simulink model "Base_Map_cs"  (R2019a)
settings: Solver=FixedStepDiscrete  StartTime=0.0  StopTime=15  FixedStep=1/300  RelTol=1e-3
PreLoadFcn:
  | mbxruntime.callbacks.PreLoadFcn(bdroot);
  | check_NUTS_defined
  | model_closed = 0;
  | assignin('base',['model_closed_' bdroot],false);
PostLoadFcn:
  | mbxruntime.callbacks.PostLoadFcn(bdroot);
InitFcn:
  | mbxruntime.callbacks.InitFcn(bdroot);
StartFcn:
  | mbxruntime.callbacks.StartFcn(bdroot);
StopFcn:
  | mbxruntime.callbacks.StopFcn(bdroot);;
  | 
model workspace: external: MAT-File .\Base_Map_S_cs_hws.mat (data not in the file)
undefined symbols (not defined in the file or in its folder): AngularVelocity, Clock_, Data, Data_SL_Info, DiscIntNeverNeededParam, Encoding, Encoding_SL_Info, Header, Height, InitImageOutputDir, LinearAcceleration, mbxruntime, Orientation, Pose, Poses, Poses_SL_Info, Position, Step, tabledata, Twist, Width
libraries: PBCSimulinkLibrary x53, robotlib x26, simulink_extras x19, PreScanSimulinkLibrary x6, dspindex x4, robotcorelib x2, sharedtransform x2, visionconversions x1, visionsinks x1
(part 4 of 8)

== system Base_Map_cs/TrafficLightRoadSideNL_5_Casing.LightOrange_Control ==
  TrafficLightRoadSideNL_5_Casing.LightOrange_Control : Inport  Tag=inport/plugin/sfun_PBCLight  OutDataTypeStr=Bus: PRESCAN_PBCLIGHT_DATA  PortDimensions=1  SampleTime=0.05  BusOutputAsStruct=on
  Actuator : S-Function  LoadFcn=addpath 'C:/Program Files/Simcenter Prescan/Prescan_2019.1/Plugins/PBCameraPlugin/matlab';addpath 'C:/Program Files/Simcenter Prescan/Prescan_2019.1/Plugins/PBCameraPlugin/bin';load('PreScanPBCLightData.mat');  FunctionName=sfun_PBCLight  Parameters=lightID, timestepMask  SFunctionDeploymentMode=off  EnableBusSupport=off  mask(Physics Based Camera plugin block){lightID=13, timestepMask=0.05}
      mask prompts: lightID "Light ID:"; timestepMask "MATLAB timestep:"
      mask help: Light Control I/O
      mask Help: eval('openHelp(6500)')
      mask Display: image(imread('ico_PBCControl.png'))
  wires:
  TrafficLightRoadSideNL_5_Casing.LightOrange_Control/1 -> Actuator/1

== system Base_Map_cs/TrafficLightRoadSideNL_5_Casing.LightRed_Control ==
  TrafficLightRoadSideNL_5_Casing.LightRed_Control : Inport  Tag=inport/plugin/sfun_PBCLight  OutDataTypeStr=Bus: PRESCAN_PBCLIGHT_DATA  PortDimensions=1  SampleTime=0.05  BusOutputAsStruct=on
  Actuator : S-Function  LoadFcn=addpath 'C:/Program Files/Simcenter Prescan/Prescan_2019.1/Plugins/PBCameraPlugin/matlab';addpath 'C:/Program Files/Simcenter Prescan/Prescan_2019.1/Plugins/PBCameraPlugin/bin';load('PreScanPBCLightData.mat');  FunctionName=sfun_PBCLight  Parameters=lightID, timestepMask  SFunctionDeploymentMode=off  EnableBusSupport=off  mask(Physics Based Camera plugin block){lightID=12, timestepMask=0.05}
      mask prompts: lightID "Light ID:"; timestepMask "MATLAB timestep:"
      mask help: Light Control I/O
      mask Help: eval('openHelp(6500)')
      mask Display: image(imread('ico_PBCControl.png'))
  wires:
  TrafficLightRoadSideNL_5_Casing.LightRed_Control/1 -> Actuator/1

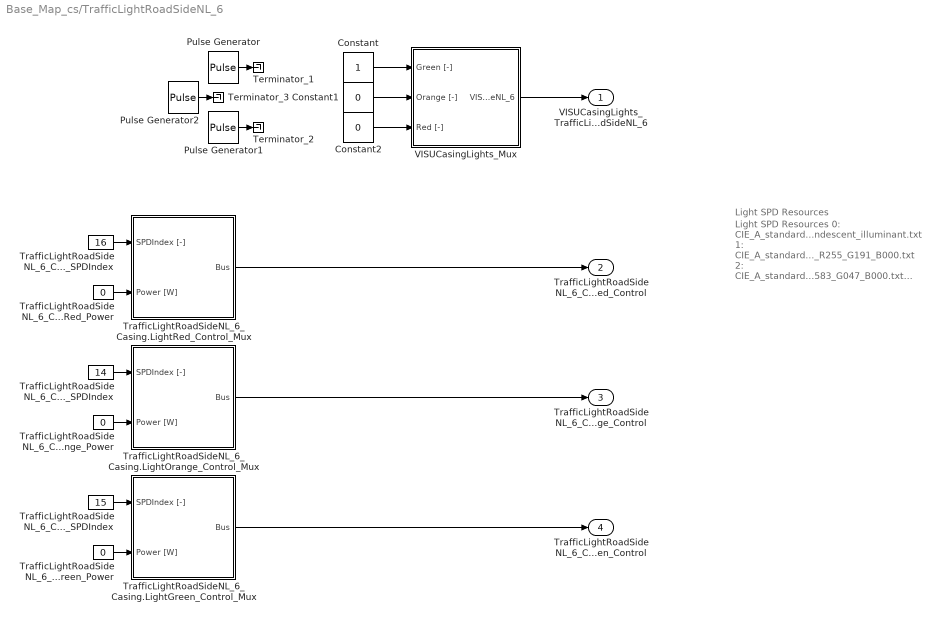
== system Base_Map_cs/TrafficLightRoadSideNL_6 ==
  note: Light SPD Resources
      |
      |  0: CIE_A_standard_incandescent_illuminant.txt
      |  1: CIE_A_standard_incandescent_illuminant.txt_x_R255_G191_B000.txt
      |  2: CIE_A_standard_incandescent_illuminant.txt_x_R583_G047_B000.txt
      |  3: CIE_F12_standard_fluorescent_illuminant.txt
      |  4: Illuminant_D65.txt
      |  5: Light_SPD_H1_12_8V_Filament.txt
      |  6: Light_SPD_H1_13_2V_Filament.txt
      |  7: Light_SPD_H11_12V_Filament.txt
      |  8: Light_SPD_H7_12_8V_Filament.txt
      |  9: Light_SPD_H7_13_2V_Filament.txt
      | 10: Light_SPD_H8_13_2V_Filament.txt
      | 11: Light_SPD_Halogen.txt
      | 12: Light_SPD_High_Power_LED.txt
      | 13: Light_SPD_HPS_High_Pressure_Sodium.txt
      | 14: Light_SPD_incandescent_traffic_signal_amber.txt
      | 15: Light_SPD_incandescent_traffic_signal_green.txt
      | 16: Light_SPD_incandescent_traffic_signal_red.txt
      | 17: Light_SPD_LED_D1S_HID.txt
      | 18: Light_SPD_LED_traffic_signal_amber.txt
      | 19: Light_SPD_LED_traffic_signal_green.txt
      | 20: Light_SPD_LED_traffic_signal_red.txt
      | 21: Light_SPD_LPS_Low_Pressure_Sodium.txt
      | 22: Light_SPD_Mercury.txt
      | 23: Light_SPD_Reddish_Neon_Sign.txt
      | 24: Noma_Twister_Blue_13W_120V.txt
      | 25: Philips_Blue_Golite_P1_Apollo_1750Lux.txt
      | 26: SPD_flat_1.0.txt
  note: Light SPD Resources
  Constant : Constant
  Constant1 : Constant  Value=0
  Constant2 : Constant  Value=0
  Pulse Generator : DiscretePulseGenerator  PulseType=Time based  Period=10  PulseWidth=40
  Pulse Generator1 : DiscretePulseGenerator  PulseType=Time based  Period=10  PulseWidth=40  PhaseDelay=6
  Pulse Generator2 : DiscretePulseGenerator  PulseType=Time based  Period=10  PulseWidth=20  PhaseDelay=4
  Terminator_1 : Terminator
  Terminator_2 : Terminator
  Terminator_3 : Terminator
  TrafficLightRoadSideNL_6_Casing.LightGreen_Control_Mux : Subsystem  Tag=mux/plugin/LightSignals
  TrafficLightRoadSideNL_6_Casing.LightGreen_Power : Constant  Tag=TrafficLightRoadSideNL_6_Casing.LightGreen_Power  Value=0
  TrafficLightRoadSideNL_6_Casing.LightGreen_SPDIndex : Constant  Tag=TrafficLightRoadSideNL_6_Casing.LightGreen_SPDIndex  Value=15
  TrafficLightRoadSideNL_6_Casing.LightOrange_Control_Mux : Subsystem  Tag=mux/plugin/LightSignals
  TrafficLightRoadSideNL_6_Casing.LightOrange_Power : Constant  Tag=TrafficLightRoadSideNL_6_Casing.LightOrange_Power  Value=0
  TrafficLightRoadSideNL_6_Casing.LightOrange_SPDIndex : Constant  Tag=TrafficLightRoadSideNL_6_Casing.LightOrange_SPDIndex  Value=14
  TrafficLightRoadSideNL_6_Casing.LightRed_Control_Mux : Subsystem  Tag=mux/plugin/LightSignals
  TrafficLightRoadSideNL_6_Casing.LightRed_Power : Constant  Tag=TrafficLightRoadSideNL_6_Casing.LightRed_Power  Value=0
  TrafficLightRoadSideNL_6_Casing.LightRed_SPDIndex : Constant  Tag=TrafficLightRoadSideNL_6_Casing.LightRed_SPDIndex  Value=16
  VISUCasingLights_Mux : Subsystem  Tag=mux/VisuCasingLights  mask(PreScan User Interface: VisuTrafficLight){}
      mask help:
      | The VisuTrafficLight block provides a way to animate traffic lights: switch on and off individual lights.
      |
      | For more information, please click Help.
      mask Help: eval('openHelp(731)')
  VISUCasingLights_TrafficLightRoadSideNL_6 : Outport  Tag=outport/VisuCasingLights  SampleTime=1/300
  TrafficLightRoadSideNL_6_Casing.LightRed_Control : Outport  Tag=outport/plugin/sfun_PBCLight  Port=2  OutDataTypeStr=Bus: PRESCAN_PBCLIGHT_DATA  PortDimensions=1  SampleTime=0.05
  TrafficLightRoadSideNL_6_Casing.LightOrange_Control : Outport  Tag=outport/plugin/sfun_PBCLight  Port=3  OutDataTypeStr=Bus: PRESCAN_PBCLIGHT_DATA  PortDimensions=1  SampleTime=0.05
  TrafficLightRoadSideNL_6_Casing.LightGreen_Control : Outport  Tag=outport/plugin/sfun_PBCLight  Port=4  OutDataTypeStr=Bus: PRESCAN_PBCLIGHT_DATA  PortDimensions=1  SampleTime=0.05
  wires:
  Constant/1 -> VISUCasingLights_Mux/1(Green [-])
  Constant1/1 -> VISUCasingLights_Mux/2(Orange [-])
  Constant2/1 -> VISUCasingLights_Mux/3(Red [-])
  VISUCasingLights_Mux/1(VISUCasingLights_TrafficLightRoadSideNL_6) -> VISUCasingLights_TrafficLightRoadSideNL_6/1
  TrafficLightRoadSideNL_6_Casing.LightRed_Control_Mux/1(Bus) -> TrafficLightRoadSideNL_6_Casing.LightRed_Control/1
  TrafficLightRoadSideNL_6_Casing.LightRed_SPDIndex/1 -> TrafficLightRoadSideNL_6_Casing.LightRed_Control_Mux/1(SPDIndex [-])
  TrafficLightRoadSideNL_6_Casing.LightRed_Power/1 -> TrafficLightRoadSideNL_6_Casing.LightRed_Control_Mux/2(Power [W])
  TrafficLightRoadSideNL_6_Casing.LightOrange_Control_Mux/1(Bus) -> TrafficLightRoadSideNL_6_Casing.LightOrange_Control/1
  TrafficLightRoadSideNL_6_Casing.LightOrange_SPDIndex/1 -> TrafficLightRoadSideNL_6_Casing.LightOrange_Control_Mux/1(SPDIndex [-])
  TrafficLightRoadSideNL_6_Casing.LightOrange_Power/1 -> TrafficLightRoadSideNL_6_Casing.LightOrange_Control_Mux/2(Power [W])
  TrafficLightRoadSideNL_6_Casing.LightGreen_Control_Mux/1(Bus) -> TrafficLightRoadSideNL_6_Casing.LightGreen_Control/1
  TrafficLightRoadSideNL_6_Casing.LightGreen_SPDIndex/1 -> TrafficLightRoadSideNL_6_Casing.LightGreen_Control_Mux/1(SPDIndex [-])
  TrafficLightRoadSideNL_6_Casing.LightGreen_Power/1 -> TrafficLightRoadSideNL_6_Casing.LightGreen_Control_Mux/2(Power [W])
  Pulse Generator/1 -> Terminator_1/1
  Pulse Generator1/1 -> Terminator_2/1
  Pulse Generator2/1 -> Terminator_3/1

== system Base_Map_cs/TrafficLightRoadSideNL_6_Casing.LightGreen_Control ==
  TrafficLightRoadSideNL_6_Casing.LightGreen_Control : Inport  Tag=inport/plugin/sfun_PBCLight  OutDataTypeStr=Bus: PRESCAN_PBCLIGHT_DATA  PortDimensions=1  SampleTime=0.05  BusOutputAsStruct=on
  Actuator : S-Function  LoadFcn=addpath 'C:/Program Files/Simcenter Prescan/Prescan_2019.1/Plugins/PBCameraPlugin/matlab';addpath 'C:/Program Files/Simcenter Prescan/Prescan_2019.1/Plugins/PBCameraPlugin/bin';load('PreScanPBCLightData.mat');  FunctionName=sfun_PBCLight  Parameters=lightID, timestepMask  SFunctionDeploymentMode=off  EnableBusSupport=off  mask(Physics Based Camera plugin block){lightID=23, timestepMask=0.05}
      mask prompts: lightID "Light ID:"; timestepMask "MATLAB timestep:"
      mask help: Light Control I/O
      mask Help: eval('openHelp(6500)')
      mask Display: image(imread('ico_PBCControl.png'))
  wires:
  TrafficLightRoadSideNL_6_Casing.LightGreen_Control/1 -> Actuator/1

== system Base_Map_cs/TrafficLightRoadSideNL_6_Casing.LightOrange_Control ==
  TrafficLightRoadSideNL_6_Casing.LightOrange_Control : Inport  Tag=inport/plugin/sfun_PBCLight  OutDataTypeStr=Bus: PRESCAN_PBCLIGHT_DATA  PortDimensions=1  SampleTime=0.05  BusOutputAsStruct=on
  Actuator : S-Function  LoadFcn=addpath 'C:/Program Files/Simcenter Prescan/Prescan_2019.1/Plugins/PBCameraPlugin/matlab';addpath 'C:/Program Files/Simcenter Prescan/Prescan_2019.1/Plugins/PBCameraPlugin/bin';load('PreScanPBCLightData.mat');  FunctionName=sfun_PBCLight  Parameters=lightID, timestepMask  SFunctionDeploymentMode=off  EnableBusSupport=off  mask(Physics Based Camera plugin block){lightID=22, timestepMask=0.05}
      mask prompts: lightID "Light ID:"; timestepMask "MATLAB timestep:"
      mask help: Light Control I/O
      mask Help: eval('openHelp(6500)')
      mask Display: image(imread('ico_PBCControl.png'))
  wires:
  TrafficLightRoadSideNL_6_Casing.LightOrange_Control/1 -> Actuator/1

== system Base_Map_cs/TrafficLightRoadSideNL_6_Casing.LightRed_Control ==
  TrafficLightRoadSideNL_6_Casing.LightRed_Control : Inport  Tag=inport/plugin/sfun_PBCLight  OutDataTypeStr=Bus: PRESCAN_PBCLIGHT_DATA  PortDimensions=1  SampleTime=0.05  BusOutputAsStruct=on
  Actuator : S-Function  LoadFcn=addpath 'C:/Program Files/Simcenter Prescan/Prescan_2019.1/Plugins/PBCameraPlugin/matlab';addpath 'C:/Program Files/Simcenter Prescan/Prescan_2019.1/Plugins/PBCameraPlugin/bin';load('PreScanPBCLightData.mat');  FunctionName=sfun_PBCLight  Parameters=lightID, timestepMask  SFunctionDeploymentMode=off  EnableBusSupport=off  mask(Physics Based Camera plugin block){lightID=21, timestepMask=0.05}
      mask prompts: lightID "Light ID:"; timestepMask "MATLAB timestep:"
      mask help: Light Control I/O
      mask Help: eval('openHelp(6500)')
      mask Display: image(imread('ico_PBCControl.png'))
  wires:
  TrafficLightRoadSideNL_6_Casing.LightRed_Control/1 -> Actuator/1

== system Base_Map_cs/TrafficLightRoadSideNL_7 ==
  note: Light SPD Resources
      |
      |  0: CIE_A_standard_incandescent_illuminant.txt
      |  1: CIE_A_standard_incandescent_illuminant.txt_x_R255_G191_B000.txt
      |  2: CIE_A_standard_incandescent_illuminant.txt_x_R583_G047_B000.txt
      |  3: CIE_F12_standard_fluorescent_illuminant.txt
      |  4: Illuminant_D65.txt
      |  5: Light_SPD_H1_12_8V_Filament.txt
      |  6: Light_SPD_H1_13_2V_Filament.txt
      |  7: Light_SPD_H11_12V_Filament.txt
      |  8: Light_SPD_H7_12_8V_Filament.txt
      |  9: Light_SPD_H7_13_2V_Filament.txt
      | 10: Light_SPD_H8_13_2V_Filament.txt
      | 11: Light_SPD_Halogen.txt
      | 12: Light_SPD_High_Power_LED.txt
      | 13: Light_SPD_HPS_High_Pressure_Sodium.txt
      | 14: Light_SPD_incandescent_traffic_signal_amber.txt
      | 15: Light_SPD_incandescent_traffic_signal_green.txt
      | 16: Light_SPD_incandescent_traffic_signal_red.txt
      | 17: Light_SPD_LED_D1S_HID.txt
      | 18: Light_SPD_LED_traffic_signal_amber.txt
      | 19: Light_SPD_LED_traffic_signal_green.txt
      | 20: Light_SPD_LED_traffic_signal_red.txt
      | 21: Light_SPD_LPS_Low_Pressure_Sodium.txt
      | 22: Light_SPD_Mercury.txt
      | 23: Light_SPD_Reddish_Neon_Sign.txt
      | 24: Noma_Twister_Blue_13W_120V.txt
      | 25: Philips_Blue_Golite_P1_Apollo_1750Lux.txt
      | 26: SPD_flat_1.0.txt
  note: Light SPD Resources
  Ground_1 : Ground
  Ground_2 : Ground
  Ground_3 : Ground
  TrafficLightRoadSideNL_7_Casing.LightGreen_Control_Mux : Subsystem  Tag=mux/plugin/LightSignals
  TrafficLightRoadSideNL_7_Casing.LightGreen_Power : Constant  Tag=TrafficLightRoadSideNL_7_Casing.LightGreen_Power  Value=0
  TrafficLightRoadSideNL_7_Casing.LightGreen_SPDIndex : Constant  Tag=TrafficLightRoadSideNL_7_Casing.LightGreen_SPDIndex  Value=15
  TrafficLightRoadSideNL_7_Casing.LightOrange_Control_Mux : Subsystem  Tag=mux/plugin/LightSignals
  TrafficLightRoadSideNL_7_Casing.LightOrange_Power : Constant  Tag=TrafficLightRoadSideNL_7_Casing.LightOrange_Power  Value=0
  TrafficLightRoadSideNL_7_Casing.LightOrange_SPDIndex : Constant  Tag=TrafficLightRoadSideNL_7_Casing.LightOrange_SPDIndex  Value=14
  TrafficLightRoadSideNL_7_Casing.LightRed_Control_Mux : Subsystem  Tag=mux/plugin/LightSignals
  TrafficLightRoadSideNL_7_Casing.LightRed_Power : Constant  Tag=TrafficLightRoadSideNL_7_Casing.LightRed_Power  Value=0
  TrafficLightRoadSideNL_7_Casing.LightRed_SPDIndex : Constant  Tag=TrafficLightRoadSideNL_7_Casing.LightRed_SPDIndex  Value=16
  VISUCasingLights_Mux : Subsystem  Tag=mux/VisuCasingLights  mask(PreScan User Interface: VisuTrafficLight){}
      mask help:
      | The VisuTrafficLight block provides a way to animate traffic lights: switch on and off individual lights.
      |
      | For more information, please click Help.
      mask Help: eval('openHelp(731)')
  VISUCasingLights_TrafficLightRoadSideNL_7 : Outport  Tag=outport/VisuCasingLights  SampleTime=1/300
  TrafficLightRoadSideNL_7_Casing.LightRed_Control : Outport  Tag=outport/plugin/sfun_PBCLight  Port=2  OutDataTypeStr=Bus: PRESCAN_PBCLIGHT_DATA  PortDimensions=1  SampleTime=0.05
  TrafficLightRoadSideNL_7_Casing.LightOrange_Control : Outport  Tag=outport/plugin/sfun_PBCLight  Port=3  OutDataTypeStr=Bus: PRESCAN_PBCLIGHT_DATA  PortDimensions=1  SampleTime=0.05
  TrafficLightRoadSideNL_7_Casing.LightGreen_Control : Outport  Tag=outport/plugin/sfun_PBCLight  Port=4  OutDataTypeStr=Bus: PRESCAN_PBCLIGHT_DATA  PortDimensions=1  SampleTime=0.05
  wires:
  VISUCasingLights_Mux/1(VISUCasingLights_TrafficLightRoadSideNL_7) -> VISUCasingLights_TrafficLightRoadSideNL_7/1
  TrafficLightRoadSideNL_7_Casing.LightRed_Control_Mux/1(Bus) -> TrafficLightRoadSideNL_7_Casing.LightRed_Control/1
  TrafficLightRoadSideNL_7_Casing.LightRed_SPDIndex/1 -> TrafficLightRoadSideNL_7_Casing.LightRed_Control_Mux/1(SPDIndex [-])
  TrafficLightRoadSideNL_7_Casing.LightRed_Power/1 -> TrafficLightRoadSideNL_7_Casing.LightRed_Control_Mux/2(Power [W])
  TrafficLightRoadSideNL_7_Casing.LightOrange_Control_Mux/1(Bus) -> TrafficLightRoadSideNL_7_Casing.LightOrange_Control/1
  TrafficLightRoadSideNL_7_Casing.LightOrange_SPDIndex/1 -> TrafficLightRoadSideNL_7_Casing.LightOrange_Control_Mux/1(SPDIndex [-])
  TrafficLightRoadSideNL_7_Casing.LightOrange_Power/1 -> TrafficLightRoadSideNL_7_Casing.LightOrange_Control_Mux/2(Power [W])
  TrafficLightRoadSideNL_7_Casing.LightGreen_Control_Mux/1(Bus) -> TrafficLightRoadSideNL_7_Casing.LightGreen_Control/1
  TrafficLightRoadSideNL_7_Casing.LightGreen_SPDIndex/1 -> TrafficLightRoadSideNL_7_Casing.LightGreen_Control_Mux/1(SPDIndex [-])
  TrafficLightRoadSideNL_7_Casing.LightGreen_Power/1 -> TrafficLightRoadSideNL_7_Casing.LightGreen_Control_Mux/2(Power [W])
  Ground_1/1 -> VISUCasingLights_Mux/1(Green [-])
  Ground_2/1 -> VISUCasingLights_Mux/2(Orange [-])
  Ground_3/1 -> VISUCasingLights_Mux/3(Red [-])

== system Base_Map_cs/TrafficLightRoadSideNL_7_Casing.LightGreen_Control ==
  TrafficLightRoadSideNL_7_Casing.LightGreen_Control : Inport  Tag=inport/plugin/sfun_PBCLight  OutDataTypeStr=Bus: PRESCAN_PBCLIGHT_DATA  PortDimensions=1  SampleTime=0.05  BusOutputAsStruct=on
  Actuator : S-Function  LoadFcn=addpath 'C:/Program Files/Simcenter Prescan/Prescan_2019.1/Plugins/PBCameraPlugin/matlab';addpath 'C:/Program Files/Simcenter Prescan/Prescan_2019.1/Plugins/PBCameraPlugin/bin';load('PreScanPBCLightData.mat');  FunctionName=sfun_PBCLight  Parameters=lightID, timestepMask  SFunctionDeploymentMode=off  EnableBusSupport=off  mask(Physics Based Camera plugin block){lightID=17, timestepMask=0.05}
      mask prompts: lightID "Light ID:"; timestepMask "MATLAB timestep:"
      mask help: Light Control I/O
      mask Help: eval('openHelp(6500)')
      mask Display: image(imread('ico_PBCControl.png'))
  wires:
  TrafficLightRoadSideNL_7_Casing.LightGreen_Control/1 -> Actuator/1

== system Base_Map_cs/TrafficLightRoadSideNL_7_Casing.LightOrange_Control ==
  TrafficLightRoadSideNL_7_Casing.LightOrange_Control : Inport  Tag=inport/plugin/sfun_PBCLight  OutDataTypeStr=Bus: PRESCAN_PBCLIGHT_DATA  PortDimensions=1  SampleTime=0.05  BusOutputAsStruct=on
  Actuator : S-Function  LoadFcn=addpath 'C:/Program Files/Simcenter Prescan/Prescan_2019.1/Plugins/PBCameraPlugin/matlab';addpath 'C:/Program Files/Simcenter Prescan/Prescan_2019.1/Plugins/PBCameraPlugin/bin';load('PreScanPBCLightData.mat');  FunctionName=sfun_PBCLight  Parameters=lightID, timestepMask  SFunctionDeploymentMode=off  EnableBusSupport=off  mask(Physics Based Camera plugin block){lightID=16, timestepMask=0.05}
      mask prompts: lightID "Light ID:"; timestepMask "MATLAB timestep:"
      mask help: Light Control I/O
      mask Help: eval('openHelp(6500)')
      mask Display: image(imread('ico_PBCControl.png'))
  wires:
  TrafficLightRoadSideNL_7_Casing.LightOrange_Control/1 -> Actuator/1

== system Base_Map_cs/TrafficLightRoadSideNL_7_Casing.LightRed_Control ==
  TrafficLightRoadSideNL_7_Casing.LightRed_Control : Inport  Tag=inport/plugin/sfun_PBCLight  OutDataTypeStr=Bus: PRESCAN_PBCLIGHT_DATA  PortDimensions=1  SampleTime=0.05  BusOutputAsStruct=on
  Actuator : S-Function  LoadFcn=addpath 'C:/Program Files/Simcenter Prescan/Prescan_2019.1/Plugins/PBCameraPlugin/matlab';addpath 'C:/Program Files/Simcenter Prescan/Prescan_2019.1/Plugins/PBCameraPlugin/bin';load('PreScanPBCLightData.mat');  FunctionName=sfun_PBCLight  Parameters=lightID, timestepMask  SFunctionDeploymentMode=off  EnableBusSupport=off  mask(Physics Based Camera plugin block){lightID=15, timestepMask=0.05}
      mask prompts: lightID "Light ID:"; timestepMask "MATLAB timestep:"
      mask help: Light Control I/O
      mask Help: eval('openHelp(6500)')
      mask Display: image(imread('ico_PBCControl.png'))
  wires:
  TrafficLightRoadSideNL_7_Casing.LightRed_Control/1 -> Actuator/1

== system Base_Map_cs/TrafficLightRoadSideNL_8 ==
  note: Light SPD Resources
      |
      |  0: CIE_A_standard_incandescent_illuminant.txt
      |  1: CIE_A_standard_incandescent_illuminant.txt_x_R255_G191_B000.txt
      |  2: CIE_A_standard_incandescent_illuminant.txt_x_R583_G047_B000.txt
      |  3: CIE_F12_standard_fluorescent_illuminant.txt
      |  4: Illuminant_D65.txt
      |  5: Light_SPD_H1_12_8V_Filament.txt
      |  6: Light_SPD_H1_13_2V_Filament.txt
      |  7: Light_SPD_H11_12V_Filament.txt
      |  8: Light_SPD_H7_12_8V_Filament.txt
      |  9: Light_SPD_H7_13_2V_Filament.txt
      | 10: Light_SPD_H8_13_2V_Filament.txt
      | 11: Light_SPD_Halogen.txt
      | 12: Light_SPD_High_Power_LED.txt
      | 13: Light_SPD_HPS_High_Pressure_Sodium.txt
      | 14: Light_SPD_incandescent_traffic_signal_amber.txt
      | 15: Light_SPD_incandescent_traffic_signal_green.txt
      | 16: Light_SPD_incandescent_traffic_signal_red.txt
      | 17: Light_SPD_LED_D1S_HID.txt
      | 18: Light_SPD_LED_traffic_signal_amber.txt
      | 19: Light_SPD_LED_traffic_signal_green.txt
      | 20: Light_SPD_LED_traffic_signal_red.txt
      | 21: Light_SPD_LPS_Low_Pressure_Sodium.txt
      | 22: Light_SPD_Mercury.txt
      | 23: Light_SPD_Reddish_Neon_Sign.txt
      | 24: Noma_Twister_Blue_13W_120V.txt
      | 25: Philips_Blue_Golite_P1_Apollo_1750Lux.txt
      | 26: SPD_flat_1.0.txt
  note: Light SPD Resources
  Ground_1 : Ground
  Ground_2 : Ground
  Ground_3 : Ground
  TrafficLightRoadSideNL_8_Casing.LightGreen_Control_Mux : Subsystem  Tag=mux/plugin/LightSignals
  TrafficLightRoadSideNL_8_Casing.LightGreen_Power : Constant  Tag=TrafficLightRoadSideNL_8_Casing.LightGreen_Power  Value=0
  TrafficLightRoadSideNL_8_Casing.LightGreen_SPDIndex : Constant  Tag=TrafficLightRoadSideNL_8_Casing.LightGreen_SPDIndex  Value=15
  TrafficLightRoadSideNL_8_Casing.LightOrange_Control_Mux : Subsystem  Tag=mux/plugin/LightSignals
  TrafficLightRoadSideNL_8_Casing.LightOrange_Power : Constant  Tag=TrafficLightRoadSideNL_8_Casing.LightOrange_Power  Value=0
  TrafficLightRoadSideNL_8_Casing.LightOrange_SPDIndex : Constant  Tag=TrafficLightRoadSideNL_8_Casing.LightOrange_SPDIndex  Value=14
  TrafficLightRoadSideNL_8_Casing.LightRed_Control_Mux : Subsystem  Tag=mux/plugin/LightSignals
  TrafficLightRoadSideNL_8_Casing.LightRed_Power : Constant  Tag=TrafficLightRoadSideNL_8_Casing.LightRed_Power  Value=0
  TrafficLightRoadSideNL_8_Casing.LightRed_SPDIndex : Constant  Tag=TrafficLightRoadSideNL_8_Casing.LightRed_SPDIndex  Value=16
  VISUCasingLights_Mux : Subsystem  Tag=mux/VisuCasingLights  mask(PreScan User Interface: VisuTrafficLight){}
      mask help:
      | The VisuTrafficLight block provides a way to animate traffic lights: switch on and off individual lights.
      |
      | For more information, please click Help.
      mask Help: eval('openHelp(731)')
  VISUCasingLights_TrafficLightRoadSideNL_8 : Outport  Tag=outport/VisuCasingLights  SampleTime=1/300
  TrafficLightRoadSideNL_8_Casing.LightRed_Control : Outport  Tag=outport/plugin/sfun_PBCLight  Port=2  OutDataTypeStr=Bus: PRESCAN_PBCLIGHT_DATA  PortDimensions=1  SampleTime=0.05
  TrafficLightRoadSideNL_8_Casing.LightOrange_Control : Outport  Tag=outport/plugin/sfun_PBCLight  Port=3  OutDataTypeStr=Bus: PRESCAN_PBCLIGHT_DATA  PortDimensions=1  SampleTime=0.05
  TrafficLightRoadSideNL_8_Casing.LightGreen_Control : Outport  Tag=outport/plugin/sfun_PBCLight  Port=4  OutDataTypeStr=Bus: PRESCAN_PBCLIGHT_DATA  PortDimensions=1  SampleTime=0.05
  wires:
  VISUCasingLights_Mux/1(VISUCasingLights_TrafficLightRoadSideNL_8) -> VISUCasingLights_TrafficLightRoadSideNL_8/1
  TrafficLightRoadSideNL_8_Casing.LightRed_Control_Mux/1(Bus) -> TrafficLightRoadSideNL_8_Casing.LightRed_Control/1
  TrafficLightRoadSideNL_8_Casing.LightRed_SPDIndex/1 -> TrafficLightRoadSideNL_8_Casing.LightRed_Control_Mux/1(SPDIndex [-])
  TrafficLightRoadSideNL_8_Casing.LightRed_Power/1 -> TrafficLightRoadSideNL_8_Casing.LightRed_Control_Mux/2(Power [W])
  TrafficLightRoadSideNL_8_Casing.LightOrange_Control_Mux/1(Bus) -> TrafficLightRoadSideNL_8_Casing.LightOrange_Control/1
  TrafficLightRoadSideNL_8_Casing.LightOrange_SPDIndex/1 -> TrafficLightRoadSideNL_8_Casing.LightOrange_Control_Mux/1(SPDIndex [-])
  TrafficLightRoadSideNL_8_Casing.LightOrange_Power/1 -> TrafficLightRoadSideNL_8_Casing.LightOrange_Control_Mux/2(Power [W])
  TrafficLightRoadSideNL_8_Casing.LightGreen_Control_Mux/1(Bus) -> TrafficLightRoadSideNL_8_Casing.LightGreen_Control/1
  TrafficLightRoadSideNL_8_Casing.LightGreen_SPDIndex/1 -> TrafficLightRoadSideNL_8_Casing.LightGreen_Control_Mux/1(SPDIndex [-])
  TrafficLightRoadSideNL_8_Casing.LightGreen_Power/1 -> TrafficLightRoadSideNL_8_Casing.LightGreen_Control_Mux/2(Power [W])
  Ground_1/1 -> VISUCasingLights_Mux/1(Green [-])
  Ground_2/1 -> VISUCasingLights_Mux/2(Orange [-])
  Ground_3/1 -> VISUCasingLights_Mux/3(Red [-])

== system Base_Map_cs/TrafficLightRoadSideNL_8_Casing.LightGreen_Control ==
  TrafficLightRoadSideNL_8_Casing.LightGreen_Control : Inport  Tag=inport/plugin/sfun_PBCLight  OutDataTypeStr=Bus: PRESCAN_PBCLIGHT_DATA  PortDimensions=1  SampleTime=0.05  BusOutputAsStruct=on
  Actuator : S-Function  LoadFcn=addpath 'C:/Program Files/Simcenter Prescan/Prescan_2019.1/Plugins/PBCameraPlugin/matlab';addpath 'C:/Program Files/Simcenter Prescan/Prescan_2019.1/Plugins/PBCameraPlugin/bin';load('PreScanPBCLightData.mat');  FunctionName=sfun_PBCLight  Parameters=lightID, timestepMask  SFunctionDeploymentMode=off  EnableBusSupport=off  mask(Physics Based Camera plugin block){lightID=20, timestepMask=0.05}
      mask prompts: lightID "Light ID:"; timestepMask "MATLAB timestep:"
      mask help: Light Control I/O
      mask Help: eval('openHelp(6500)')
      mask Display: image(imread('ico_PBCControl.png'))
  wires:
  TrafficLightRoadSideNL_8_Casing.LightGreen_Control/1 -> Actuator/1

== system Base_Map_cs/TrafficLightRoadSideNL_8_Casing.LightOrange_Control ==
  TrafficLightRoadSideNL_8_Casing.LightOrange_Control : Inport  Tag=inport/plugin/sfun_PBCLight  OutDataTypeStr=Bus: PRESCAN_PBCLIGHT_DATA  PortDimensions=1  SampleTime=0.05  BusOutputAsStruct=on
  Actuator : S-Function  LoadFcn=addpath 'C:/Program Files/Simcenter Prescan/Prescan_2019.1/Plugins/PBCameraPlugin/matlab';addpath 'C:/Program Files/Simcenter Prescan/Prescan_2019.1/Plugins/PBCameraPlugin/bin';load('PreScanPBCLightData.mat');  FunctionName=sfun_PBCLight  Parameters=lightID, timestepMask  SFunctionDeploymentMode=off  EnableBusSupport=off  mask(Physics Based Camera plugin block){lightID=19, timestepMask=0.05}
      mask prompts: lightID "Light ID:"; timestepMask "MATLAB timestep:"
      mask help: Light Control I/O
      mask Help: eval('openHelp(6500)')
      mask Display: image(imread('ico_PBCControl.png'))
  wires:
  TrafficLightRoadSideNL_8_Casing.LightOrange_Control/1 -> Actuator/1

== system Base_Map_cs/TrafficLightRoadSideNL_8_Casing.LightRed_Control ==
  TrafficLightRoadSideNL_8_Casing.LightRed_Control : Inport  Tag=inport/plugin/sfun_PBCLight  OutDataTypeStr=Bus: PRESCAN_PBCLIGHT_DATA  PortDimensions=1  SampleTime=0.05  BusOutputAsStruct=on
  Actuator : S-Function  LoadFcn=addpath 'C:/Program Files/Simcenter Prescan/Prescan_2019.1/Plugins/PBCameraPlugin/matlab';addpath 'C:/Program Files/Simcenter Prescan/Prescan_2019.1/Plugins/PBCameraPlugin/bin';load('PreScanPBCLightData.mat');  FunctionName=sfun_PBCLight  Parameters=lightID, timestepMask  SFunctionDeploymentMode=off  EnableBusSupport=off  mask(Physics Based Camera plugin block){lightID=18, timestepMask=0.05}
      mask prompts: lightID "Light ID:"; timestepMask "MATLAB timestep:"
      mask help: Light Control I/O
      mask Help: eval('openHelp(6500)')
      mask Display: image(imread('ico_PBCControl.png'))
  wires:
  TrafficLightRoadSideNL_8_Casing.LightRed_Control/1 -> Actuator/1

== system Base_Map_cs/VISUCasingLights_TrafficLightRoadSideNL_1 ==
  VISUCasingLights_TrafficLightRoadSideNL_1 : Inport  Tag=inport/VisuCasingLights  SampleTime=1/300  BusOutputAsStruct=on
  Actuator : Subsystem  mask(PreScan Sink Block: VisuTrafficLight){UniqueID=646, ColorsObjectQuery=, Colors=[]}
      mask prompts: UniqueID "Parent Unique Identifier"; ColorsObjectQuery "Query for Color Object"; Colors "Matrix of colors"
      mask help:
      | The VisuTrafficLight block provides a way to animate traffic lights: switch on and off individual lights.
      |
      | For more information, please click Help.
      mask Help: eval('openHelp(731)')
      mask Display: image(imread('TrafficLightCasing.png'))
  wires:
  VISUCasingLights_TrafficLightRoadSideNL_1/1 -> Actuator/1(VISUCasingLights_TrafficLightRoadSideNL_1)

== system Base_Map_cs/VISUCasingLights_TrafficLightRoadSideNL_2 ==
  VISUCasingLights_TrafficLightRoadSideNL_2 : Inport  Tag=inport/VisuCasingLights  SampleTime=1/300  BusOutputAsStruct=on
  Actuator : Subsystem  mask(PreScan Sink Block: VisuTrafficLight){UniqueID=647, ColorsObjectQuery=, Colors=[]}
      mask prompts: UniqueID "Parent Unique Identifier"; ColorsObjectQuery "Query for Color Object"; Colors "Matrix of colors"
      mask help:
      | The VisuTrafficLight block provides a way to animate traffic lights: switch on and off individual lights.
      |
      | For more information, please click Help.
      mask Help: eval('openHelp(731)')
      mask Display: image(imread('TrafficLightCasing.png'))
  wires:
  VISUCasingLights_TrafficLightRoadSideNL_2/1 -> Actuator/1(VISUCasingLights_TrafficLightRoadSideNL_2)

== system Base_Map_cs/VISUCasingLights_TrafficLightRoadSideNL_3 ==
  VISUCasingLights_TrafficLightRoadSideNL_3 : Inport  Tag=inport/VisuCasingLights  SampleTime=1/300  BusOutputAsStruct=on
  Actuator : Subsystem  mask(PreScan Sink Block: VisuTrafficLight){UniqueID=649, ColorsObjectQuery=, Colors=[]}
      mask prompts: UniqueID "Parent Unique Identifier"; ColorsObjectQuery "Query for Color Object"; Colors "Matrix of colors"
      mask help:
      | The VisuTrafficLight block provides a way to animate traffic lights: switch on and off individual lights.
      |
      | For more information, please click Help.
      mask Help: eval('openHelp(731)')
      mask Display: image(imread('TrafficLightCasing.png'))
  wires:
  VISUCasingLights_TrafficLightRoadSideNL_3/1 -> Actuator/1(VISUCasingLights_TrafficLightRoadSideNL_3)

== system Base_Map_cs/VISUCasingLights_TrafficLightRoadSideNL_4 ==
  VISUCasingLights_TrafficLightRoadSideNL_4 : Inport  Tag=inport/VisuCasingLights  SampleTime=1/300  BusOutputAsStruct=on
  Actuator : Subsystem  mask(PreScan Sink Block: VisuTrafficLight){UniqueID=650, ColorsObjectQuery=, Colors=[]}
      mask prompts: UniqueID "Parent Unique Identifier"; ColorsObjectQuery "Query for Color Object"; Colors "Matrix of colors"
      mask help:
      | The VisuTrafficLight block provides a way to animate traffic lights: switch on and off individual lights.
      |
      | For more information, please click Help.
      mask Help: eval('openHelp(731)')
      mask Display: image(imread('TrafficLightCasing.png'))
  wires:
  VISUCasingLights_TrafficLightRoadSideNL_4/1 -> Actuator/1(VISUCasingLights_TrafficLightRoadSideNL_4)

== system Base_Map_cs/VISUCasingLights_TrafficLightRoadSideNL_5 ==
  VISUCasingLights_TrafficLightRoadSideNL_5 : Inport  Tag=inport/VisuCasingLights  SampleTime=1/300  BusOutputAsStruct=on
  Actuator : Subsystem  mask(PreScan Sink Block: VisuTrafficLight){UniqueID=651, ColorsObjectQuery=, Colors=[]}
      mask prompts: UniqueID "Parent Unique Identifier"; ColorsObjectQuery "Query for Color Object"; Colors "Matrix of colors"
      mask help:
      | The VisuTrafficLight block provides a way to animate traffic lights: switch on and off individual lights.
      |
      | For more information, please click Help.
      mask Help: eval('openHelp(731)')
      mask Display: image(imread('TrafficLightCasing.png'))
  wires:
  VISUCasingLights_TrafficLightRoadSideNL_5/1 -> Actuator/1(VISUCasingLights_TrafficLightRoadSideNL_5)

== system Base_Map_cs/VISUCasingLights_TrafficLightRoadSideNL_6 ==
  VISUCasingLights_TrafficLightRoadSideNL_6 : Inport  Tag=inport/VisuCasingLights  SampleTime=1/300  BusOutputAsStruct=on
  Actuator : Subsystem  mask(PreScan Sink Block: VisuTrafficLight){UniqueID=10446, ColorsObjectQuery=, Colors=[]}
      mask prompts: UniqueID "Parent Unique Identifier"; ColorsObjectQuery "Query for Color Object"; Colors "Matrix of colors"
      mask help:
      | The VisuTrafficLight block provides a way to animate traffic lights: switch on and off individual lights.
      |
      | For more information, please click Help.
      mask Help: eval('openHelp(731)')
      mask Display: image(imread('TrafficLightCasing.png'))
  wires:
  VISUCasingLights_TrafficLightRoadSideNL_6/1 -> Actuator/1(VISUCasingLights_TrafficLightRoadSideNL_6)

== system Base_Map_cs/VISUCasingLights_TrafficLightRoadSideNL_7 ==
  VISUCasingLights_TrafficLightRoadSideNL_7 : Inport  Tag=inport/VisuCasingLights  SampleTime=1/300  BusOutputAsStruct=on
  Actuator : Subsystem  mask(PreScan Sink Block: VisuTrafficLight){UniqueID=653, ColorsObjectQuery=, Colors=[]}
      mask prompts: UniqueID "Parent Unique Identifier"; ColorsObjectQuery "Query for Color Object"; Colors "Matrix of colors"
      mask help:
      | The VisuTrafficLight block provides a way to animate traffic lights: switch on and off individual lights.
      |
      | For more information, please click Help.
      mask Help: eval('openHelp(731)')
      mask Display: image(imread('TrafficLightCasing.png'))
  wires:
  VISUCasingLights_TrafficLightRoadSideNL_7/1 -> Actuator/1(VISUCasingLights_TrafficLightRoadSideNL_7)

== system Base_Map_cs/VISUCasingLights_TrafficLightRoadSideNL_8 ==
  VISUCasingLights_TrafficLightRoadSideNL_8 : Inport  Tag=inport/VisuCasingLights  SampleTime=1/300  BusOutputAsStruct=on
  Actuator : Subsystem  mask(PreScan Sink Block: VisuTrafficLight){UniqueID=654, ColorsObjectQuery=, Colors=[]}
      mask prompts: UniqueID "Parent Unique Identifier"; ColorsObjectQuery "Query for Color Object"; Colors "Matrix of colors"
      mask help:
      | The VisuTrafficLight block provides a way to animate traffic lights: switch on and off individual lights.
      |
      | For more information, please click Help.
      mask Help: eval('openHelp(731)')
      mask Display: image(imread('TrafficLightCasing.png'))
  wires:
  VISUCasingLights_TrafficLightRoadSideNL_8/1 -> Actuator/1(VISUCasingLights_TrafficLightRoadSideNL_8)

== system Base_Map_cs/camera ==
  Sensor : S-Function  FunctionName=sfun_Camera  Parameters=sensorID, dataWidth, dataHeight, channelsPerImage, numberOfImages, timestep  SFunctionDeploymentMode=off  EnableBusSupport=off  mask(PreScan Source Block: Camera Sensor){sensorID=9056, dataWidth=720, dataHeight=2880, channelsPerImage=3, numberOfImages=1, timestep=1/20}
      mask prompts: sensorID "Sensor ID"; dataWidth "Data width"; dataHeight "Data Height"; channelsPerImage "Channels per image"; numberOfImages "Number of images"; timestep "MATLAB timestep:"
      mask help: The Camera Sensor provides a color or monochrome image.
      mask Help: eval('openHelp(457)')
      mask Display: image(imread('CameraSensor.png'))
  camera : Outport  Tag=outport/Camera/CameraSensor  OutDataTypeStr=uint8  SampleTime=1/20
  wires:
  Sensor/1 -> camera/1

== system Base_Map_cs/pose_otheCar ==
  In1 : Inport
  Enable : EnablePort
  Add5 : Sum
  Assignment : Assignment  OutputInitialize=Specify size for each dimension in table  DiagnosticForDimensions=Warning  IndexOptions=Starting index (dialog)  Indices=1  OutputSizes=1
  Assignment2 : Assignment  OutputInitialize=Specify size for each dimension in table  DiagnosticForDimensions=Warning  IndexOptions=Starting index (dialog)  Indices=1  OutputSizes=1000
  Blank Message1 : robotlib/Blank Message  messageClass=Message  entityType=geometry_msgs/PoseArray  messageType=geometry_msgs/PoseArray  SampleTime=inf
      settings: SourceProductBaseCode=RO
  Bus Assignment3 : BusAssignment  AssignedSignals=Header.Seq,Header.FrameId,Header.FrameId_SL_Info.CurrentLength,Poses,Poses_SL_Info.CurrentLength
  Bus Selector : BusSelector  OutputSignals=Poses
  Bus Selector2 : BusSelector  OutputSignals=Header.FrameId
  Constant24 : Constant  OutDataTypeStr=uint32
  Constant25 : Constant  Value=uint8(['map'])
  Memory2 : Memory  InheritSampleTime=on
  Publish2 : robotlib/Publish  topicSource=Specify your own  topic=/pose_otherCar  messageType=geometry_msgs/PoseArray  messageQueueLength=1
      settings: SourceProductBaseCode=RO
  Width : Width  DataType=uint32
  Width5 : Width  DataType=uint32
  wires:
  Blank Message1/1 -> Bus Assignment3/1, Bus Selector2/1, Bus Selector/1
  Bus Selector2/1 -> Assignment2/1  "<FrameId>"
  Assignment2/1 -> Width5/1, Bus Assignment3/3
  Constant25/1 -> Assignment2/2
  Bus Assignment3/1 -> Publish2/1
  In1/1 -> Assignment/2
  Bus Selector/1 -> Assignment/1  "<Poses>"
  Width/1 -> Bus Assignment3/6
  Assignment/1 -> Width/1, Bus Assignment3/5
  Width5/1 -> Bus Assignment3/4
  Add5/1 -> Memory2/1, Bus Assignment3/2
  Memory2/1 -> Add5/1
  Constant24/1 -> Add5/2

== system Base_Map_cs/tl_camera ==
  Sensor : S-Function  FunctionName=sfun_Camera  Parameters=sensorID, dataWidth, dataHeight, channelsPerImage, numberOfImages, timestep  SFunctionDeploymentMode=off  EnableBusSupport=off  mask(PreScan Source Block: Camera Sensor){sensorID=12017, dataWidth=720, dataHeight=2880, channelsPerImage=3, numberOfImages=1, timestep=1/20}
      mask prompts: sensorID "Sensor ID"; dataWidth "Data width"; dataHeight "Data Height"; channelsPerImage "Channels per image"; numberOfImages "Number of images"; timestep "MATLAB timestep:"
      mask help: The Camera Sensor provides a color or monochrome image.
      mask Help: eval('openHelp(457)')
      mask Display: image(imread('CameraSensor.png'))
  tl_camera : Outport  Tag=outport/Camera/CameraSensor  OutDataTypeStr=uint8  SampleTime=1/20
  wires:
  Sensor/1 -> tl_camera/1

== system Base_Map_cs/BMW_X5_SUV_1/Car_Pose ==
  In1 : Inport
  In2 : Inport  Port=2
  In3 : Inport  Port=3
  In4 : Inport  Port=4
  In5 : Inport  Port=5
  In6 : Inport  Port=6
  Coordinate Transformation Conversion : robotcorelib/Coordinate Transformation Conversion  InputRepresentation=Euler Angles  InputEulerSequence=XYZ  ShowTrVecInputPort=on  OutputRepresentation=Quaternion  OutputEulerSequence=ZYX  ShowTrVecOutputPort=on  SimulateUsing=Interpreted execution
      settings: SourceProductBaseCode=RO
  Data Type Conversion : DataTypeConversion
  Data Type Conversion1 : DataTypeConversion
  Data Type Conversion2 : DataTypeConversion
  Degrees to Radians1 : simulink_extras/Transformations/Degrees to Radians
  Degrees to Radians2 : simulink_extras/Transformations/Degrees to Radians
  Degrees to Radians5 : simulink_extras/Transformations/Degrees to Radians
  Mux : Mux
  Vector Concatenate2 : Concatenate  NumInputs=3
  Out1 : Outport
  wires:
  Degrees to Radians1/1 -> Vector Concatenate2/2
  Degrees to Radians5/1 -> Vector Concatenate2/1
  Vector Concatenate2/1 -> Coordinate Transformation Conversion/1
  Degrees to Radians2/1 -> Vector Concatenate2/3
  In1/1 -> Data Type Conversion/1
  In2/1 -> Data Type Conversion1/1
  In3/1 -> Data Type Conversion2/1
  In4/1 -> Degrees to Radians5/1
  In5/1 -> Degrees to Radians1/1
  In6/1 -> Degrees to Radians2/1
  Data Type Conversion/1 -> Mux/1
  Data Type Conversion1/1 -> Mux/2
  Data Type Conversion2/1 -> Mux/3
  Coordinate Transformation Conversion/1 -> Mux/4
  Mux/1 -> Out1/1

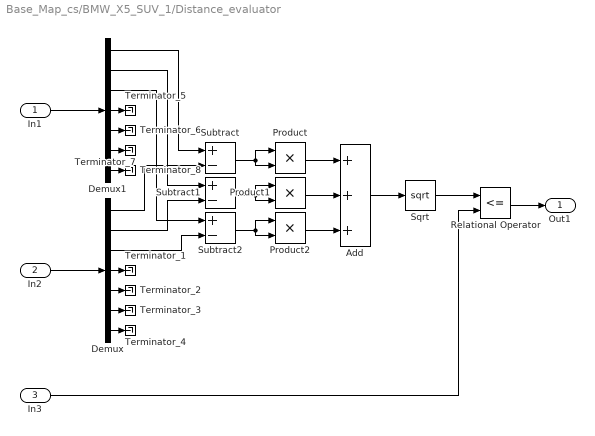
== system Base_Map_cs/BMW_X5_SUV_1/Distance_evaluator ==
  In1 : Inport
  In2 : Inport  Port=2
  In3 : Inport  Port=3
  Add : Sum  Inputs=3
  Demux : Demux  Outputs=7
  Demux1 : Demux  Outputs=7
  Product : Product
  Product1 : Product
  Product2 : Product
  Relational Operator : RelationalOperator  Operator=<=  OutDataTypeStr=boolean  RndMeth=Simplest
  Sqrt : Sqrt  SaturateOnIntegerOverflow=on
  Subtract : Sum  Inputs=+-
  Subtract1 : Sum  Inputs=+-
  Subtract2 : Sum  Inputs=+-
  Terminator_{1..8} (8 alike) : Terminator
  Out1 : Outport
  wires:
  Relational Operator/1 -> Out1/1
  In1/1 -> Demux1/1
  In2/1 -> Demux/1
  Demux1/1 -> Subtract/1
  Demux1/2 -> Subtract1/1
  Demux1/3 -> Subtract2/1
  Demux/1 -> Subtract/2
  Demux/2 -> Subtract1/2
  Demux/3 -> Subtract2/2
  Subtract/1 -> Product/1, Product/2
  Subtract1/1 -> Product1/1, Product1/2
  Subtract2/1 -> Product2/1, Product2/2
  Product/1 -> Add/1
  Product1/1 -> Add/2
  Product2/1 -> Add/3
  Add/1 -> Sqrt/1
  Sqrt/1 -> Relational Operator/1
  In3/1 -> Relational Operator/2
  Demux/4 -> Terminator_1/1
  Demux/5 -> Terminator_2/1
  Demux/6 -> Terminator_3/1
  Demux/7 -> Terminator_4/1
  Demux1/4 -> Terminator_5/1
  Demux1/5 -> Terminator_6/1
  Demux1/6 -> Terminator_7/1
  Demux1/7 -> Terminator_8/1

== system Base_Map_cs/BMW_X5_SUV_1/Dynamics_Empty ==
  note: For state mode 'Dynamic' positions
      | are not taken into account, as they
      | are computed by integrating velocity.
      | Click annotation for Help.
  Bus Selector : BusSelector  OutputSignals=Twist.Linear.X,Twist.Linear.Y,Twist.Linear.Z,Twist.Angular.X,Twist.Angular.Y,Twist.Angular.Z
  Data Type Conversion{,1..5} (6 alike) : DataTypeConversion
  Discrete-Time Integrator1 : DiscreteIntegrator  SampleTime=-1  ICPrevOutput=DiscIntNeverNeededParam  ICPrevScaledInput=DiscIntNeverNeededParam
  Discrete-Time Integrator2 : DiscreteIntegrator  SampleTime=-1  ICPrevOutput=DiscIntNeverNeededParam  ICPrevScaledInput=DiscIntNeverNeededParam
  Discrete-Time Integrator3 : DiscreteIntegrator  SampleTime=-1  ICPrevOutput=DiscIntNeverNeededParam  ICPrevScaledInput=DiscIntNeverNeededParam
  Ground_1 : Ground
  Ground_2 : Ground
  Ground_3 : Ground
  MuxState : Subsystem  Tag=mux/State  mask(Empty Dynamics State Block){positioningmode=off, TimeStep=1/300}
      mask prompts: positioningmode "Positioning Mode"; TimeStep "Auto Assigned: Time Step [s]"
      mask help:
      | Build the state of an actor based on user input.
      | The user can either use positioning mode or dynamics mode.
      | - When using positioning mode the position and orientation of the actor are set directly based on the input. Expected input is relative to the initial position and orientation of the actor. It's also possible to specify the velocity of the actor, though this input isn't used, only passed on.
      | - When using dynamics mode the position input is ignored. Expected input is velocity and orientation. The velocity is relative the current orientation of the actor, while orientation is relative to its initial orientation. The position of the actor is calculated based on the velocity and orientation given.
      settings: DeleteFcn=PreScanBlockDeleteFcn;
  STATE_BMW_X5_SUV_1 : Subsystem  Tag=mux/StatePort  Priority=0  LoadFcn=load PrescanStateActuatorData  mask(PreScan Sink Block: State){x0=26.6104, y0=171.2152, z0=0.69, Roll0=0, Pitch0=0, Yaw0=0.26655, TimeStep=1/300}
      mask prompts: x0 "Ini x-position VEHICLE wrt GLOBAL axis system [m]"; y0 "Ini y-position VEHICLE wrt GLOBAL axis system [m]"; z0 "Ini z-position VEHICLE wrt GLOBAL axis system [m]"; Roll0 "Ini roll-angle BODY wrt VEHICLE axis system [deg]"; Pitch0 "Ini pitch-angle BODY wrt VEHICLE axis system [deg]"; Yaw0 "Ini yaw-angle VEHICLE wrt GLOBAL axis system [deg]"; TimeStep "Auto-Assigned: Upload Period [s]"
      mask help:
      | The Actor State contains a vector signal of size (9x1), containing the following signals:
      |
      | -  Position                  (x,y,z)                                     [m]
      | -  Velocity                  (vx,vy,vz)                               [m/s]
      | -  Angles                    (Roll, Pitch, Yaw)                   [rad]
      |
      | The Actor state is defined in the global axis system.
      | The state is superponed on the Initial position defined in the GUI.
      |
      | For more information, please click Help.
      settings: DeleteFcn=PreScanBlockDeleteFcn;
      mask Help: eval('openHelp(222)')
      mask Display: image(imread('State.png'))
  Scope : Scope
  Sine Wave Function : Sin  Amplitude=0.1  SampleTime=0
  Subscribe : robotlib/Subscribe  topicSource=Select from ROS network  topic=/TwistS  messageType=geometry_msgs/TwistStamped  sampleTime=-1  messageQueueLength=1
      settings: SourceProductBaseCode=RO
  Terminator_1 : Terminator
  Terminator_2 : Terminator
  State : Outport  Tag=outport/StateOutport  SampleTime=1/300
  tag scope: x_speed=global
  wires:
  Bus Selector/1 -> Data Type Conversion/1, Scope/1  "<X>"
  Bus Selector/2 -> Data Type Conversion1/1  "<Y>"
  Bus Selector/3 -> Data Type Conversion2/1  "<Z>"
  Bus Selector/4 -> Data Type Conversion3/1  "<X>"
  Data Type Conversion3/1 -> Discrete-Time Integrator3/1
  Bus Selector/5 -> Data Type Conversion4/1  "<Y>"
  Data Type Conversion4/1 -> Discrete-Time Integrator2/1
  Bus Selector/6 -> Data Type Conversion5/1  "<Z>"
  Data Type Conversion5/1 -> Discrete-Time Integrator1/1
  Subscribe/2 -> Bus Selector/1
  Data Type Conversion/1 -> [x_speed], MuxState/4(dx [m/s])
  Data Type Conversion1/1 -> MuxState/5(dy [m/s])
  Data Type Conversion2/1 -> MuxState/6(dz [m/s])
  Discrete-Time Integrator3/1 -> MuxState/7(R [rad])
  Discrete-Time Integrator2/1 -> MuxState/8(P [rad])
  Discrete-Time Integrator1/1 -> MuxState/9(Y [rad])
  MuxState/1(state) -> STATE_BMW_X5_SUV_1/1(State)
  STATE_BMW_X5_SUV_1/1(StateBus) -> State/1
  Ground_1/1 -> MuxState/1(x [m])
  Ground_2/1 -> MuxState/2(y [m])
  Ground_3/1 -> MuxState/3(z [m])
  Sine Wave Function/1 -> Terminator_1/1
  Subscribe/1 -> Terminator_2/1

== system Base_Map_cs/BMW_X5_SUV_1/Frequency evaluator ==
  In1 : Inport
  Add : Sum  Inputs=+-
  Clock2 : Clock
  Constant : Constant
  Divide : Product  Inputs=*/
  Memory : Memory
  Relational Operator : RelationalOperator  OutDataTypeStr=boolean  RndMeth=Simplest
  Switch : Switch  Criteria=u2 > Threshold
  Out1 : Outport
  wires:
  Memory/1 -> Switch/3, Add/2
  Switch/1 -> Memory/1
  Add/1 -> Relational Operator/1
  Relational Operator/1 -> Switch/2, Out1/1
  Clock2/1 -> Add/1, Switch/1
  In1/1 -> Divide/2
  Constant/1 -> Divide/1
  Divide/1 -> Relational Operator/2

== system Base_Map_cs/BMW_X5_SUV_1/Frequency evaluator1 ==
  In1 : Inport
  Add : Sum  Inputs=+-
  Clock2 : Clock
  Constant : Constant
  Divide : Product  Inputs=*/
  Memory : Memory
  Relational Operator : RelationalOperator  OutDataTypeStr=boolean  RndMeth=Simplest
  Switch : Switch  Criteria=u2 > Threshold
  Out1 : Outport
  wires:
  Memory/1 -> Switch/3, Add/2
  Switch/1 -> Memory/1
  Add/1 -> Relational Operator/1
  Relational Operator/1 -> Switch/2, Out1/1
  Clock2/1 -> Add/1, Switch/1
  In1/1 -> Divide/2
  Constant/1 -> Divide/1
  Divide/1 -> Relational Operator/2

== system Base_Map_cs/BMW_X5_SUV_1/Frequency evaluator2 ==
  In1 : Inport
  Add : Sum  Inputs=+-
  Clock2 : Clock
  Constant : Constant
  Divide : Product  Inputs=*/
  Memory : Memory
  Relational Operator : RelationalOperator  OutDataTypeStr=boolean  RndMeth=Simplest
  Switch : Switch  Criteria=u2 > Threshold
  Out1 : Outport
  wires:
  Memory/1 -> Switch/3, Add/2
  Switch/1 -> Memory/1
  Add/1 -> Relational Operator/1
  Relational Operator/1 -> Switch/2, Out1/1
  Clock2/1 -> Add/1, Switch/1
  In1/1 -> Divide/2
  Constant/1 -> Divide/1
  Divide/1 -> Relational Operator/2

== system Base_Map_cs/BMW_X5_SUV_1/Frequency evaluator3 ==
  In1 : Inport
  Add : Sum  Inputs=+-
  Clock2 : Clock
  Constant : Constant
  Divide : Product  Inputs=*/
  Memory : Memory
  Relational Operator : RelationalOperator  OutDataTypeStr=boolean  RndMeth=Simplest
  Switch : Switch  Criteria=u2 > Threshold
  Out1 : Outport
  wires:
  Memory/1 -> Switch/3, Add/2
  Switch/1 -> Memory/1
  Add/1 -> Relational Operator/1
  Relational Operator/1 -> Switch/2, Out1/1
  Clock2/1 -> Add/1, Switch/1
  In1/1 -> Divide/2
  Constant/1 -> Divide/1
  Divide/1 -> Relational Operator/2

== system Base_Map_cs/BMW_X5_SUV_1/Frequency evaluator4 ==
  In1 : Inport
  Add : Sum  Inputs=+-
  Clock2 : Clock
  Constant : Constant
  Divide : Product  Inputs=*/
  Memory : Memory
  Relational Operator : RelationalOperator  OutDataTypeStr=boolean  RndMeth=Simplest
  Switch : Switch  Criteria=u2 > Threshold
  Out1 : Outport
  wires:
  Memory/1 -> Switch/3, Add/2
  Switch/1 -> Memory/1
  Add/1 -> Relational Operator/1
  Relational Operator/1 -> Switch/2, Out1/1
  Clock2/1 -> Add/1, Switch/1
  In1/1 -> Divide/2
  Constant/1 -> Divide/1
  Divide/1 -> Relational Operator/2

== system Base_Map_cs/BMW_X5_SUV_1/Frequency evaluator5 ==
  In1 : Inport
  Add : Sum  Inputs=+-
  Clock2 : Clock
  Constant : Constant
  Divide : Product  Inputs=*/
  Memory : Memory
  Relational Operator : RelationalOperator  OutDataTypeStr=boolean  RndMeth=Simplest
  Switch : Switch  Criteria=u2 > Threshold
  Out1 : Outport
  wires:
  Memory/1 -> Switch/3, Add/2
  Switch/1 -> Memory/1
  Add/1 -> Relational Operator/1
  Relational Operator/1 -> Switch/2, Out1/1
  Clock2/1 -> Add/1, Switch/1
  In1/1 -> Divide/2
  Constant/1 -> Divide/1
  Divide/1 -> Relational Operator/2

== system Base_Map_cs/BMW_X5_SUV_1/Frequency evaluator6 ==
  In1 : Inport
  Add : Sum  Inputs=+-
  Clock2 : Clock
  Constant : Constant
  Divide : Product  Inputs=*/
  Memory : Memory
  Relational Operator : RelationalOperator  OutDataTypeStr=boolean  RndMeth=Simplest
  Switch : Switch  Criteria=u2 > Threshold
  Out1 : Outport
  wires:
  Divide/1 -> Relational Operator/2
  Constant/1 -> Divide/1
  In1/1 -> Divide/2
  Clock2/1 -> Switch/1, Add/1
  Relational Operator/1 -> Out1/1, Switch/2
  Add/1 -> Relational Operator/1
  Switch/1 -> Memory/1
  Memory/1 -> Add/2, Switch/3

== system Base_Map_cs/BMW_X5_SUV_1/Frequency evaluator7 ==
  In1 : Inport
  Add : Sum  Inputs=+-
  Clock2 : Clock
  Constant : Constant
  Divide : Product  Inputs=*/
  Memory : Memory
  Relational Operator : RelationalOperator  OutDataTypeStr=boolean  RndMeth=Simplest
  Switch : Switch  Criteria=u2 > Threshold
  Out1 : Outport
  wires:
  Divide/1 -> Relational Operator/2
  Constant/1 -> Divide/1
  In1/1 -> Divide/2
  Clock2/1 -> Switch/1, Add/1
  Relational Operator/1 -> Out1/1, Switch/2
  Add/1 -> Relational Operator/1
  Switch/1 -> Memory/1
  Memory/1 -> Add/2, Switch/3

== system Base_Map_cs/BMW_X5_SUV_1/HumViewCamera_CM_Demux ==
  In1 : Inport
  Selector : Selector  NumberOfDimensions=2  InputPortWidth=3  IndexOptions=Index vector (dialog),Index vector (dialog)  Indices=-1,1:hres  OutputSizes=1,1
  Selector1 : Selector  NumberOfDimensions=2  InputPortWidth=3  IndexOptions=Index vector (dialog),Index vector (dialog)  Indices=-1,hres+1:hres*2  OutputSizes=1,1
  Selector2 : Selector  NumberOfDimensions=2  InputPortWidth=3  IndexOptions=Index vector (dialog),Index vector (dialog)  Indices=-1,hres*2+1:hres*3  OutputSizes=1,1
  R : Outport
  G : Outport  Port=2
  B : Outport  Port=3
  wires:
  In1/1 -> Selector1/1, Selector/1, Selector2/1
  Selector/1 -> R/1
  Selector1/1 -> G/1
  Selector2/1 -> B/1
